simulink model "dB_lookup_table_sim"  (R2020b)
settings: Solver=VariableStepAuto  StartTime=0.0  StopTime=stop_time  RelTol=1e-3
InitFcn:
  | dB_lookup_table_sim_init
StopFcn:
  | dB_lookup_table_sim_stop
values from neighbouring files (symbols this model uses):
  fs = 48000    [dB_lookup_table_sim_init.m]
libraries: dspsrcs4 x1
settings Model: Creator=t96f346  LastModifiedBy=conno
settings DataIOCC: ReturnWorkspaceOutputs=off
settings OptimizationCC: BlockReduction=off  ConditionallyExecuteInputs=off  DefaultParameterBehavior=Inlined

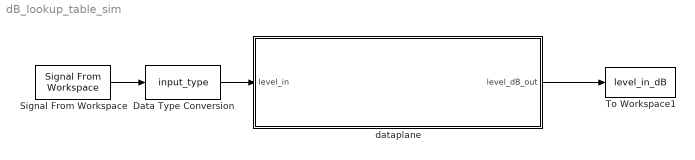
== system dB_lookup_table_sim ==
  Data Type Conversion : DataTypeConversion  OutDataTypeStr=input_type
  Signal From Workspace : dspsrcs4/Signal From Workspace  X=level_in  Ts=1/fs  nsamps=1  OutputAfterFinalValue=Setting to zero  ignoreOrWarnInputAndFrameLengths=off  OutputFrames=off
  To Workspace1 : ToWorkspace  VariableName=level_in_dB  SampleTime=-1
      settings: Save2DSignal=2-D array (concatenate along first dimension)
  dataplane : Subsystem
  wires:
  Signal From Workspace/1 -> Data Type Conversion/1
  Data Type Conversion/1 -> dataplane/1(level_in)
  dataplane/1(level_dB_out) -> To Workspace1/1

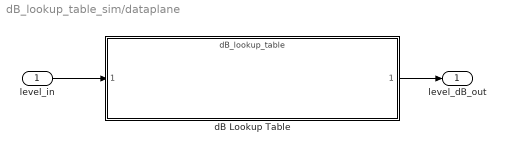
== system dB_lookup_table_sim/dataplane ==
  level_in : Inport
  dB Lookup Table : ModelReference  ModelNameDialog=dB_lookup_table  SimulationMode=Normal  ModelReferenceVersion=2.65
  level_dB_out : Outport
  wires:
  level_in/1 -> dB Lookup Table/1
  dB Lookup Table/1 -> level_dB_out/1
